simulink model "realimentacao_estados"  (R2022b)
settings: Solver=VariableStepAuto  StartTime=0.0  StopTime=30  RelTol=1e-3
values from neighbouring files (symbols this model uses):
  Cd = ss_d.C    [espacoDiscreto.m]
  Dd = ss_d.D    [espacoDiscreto.m]
  disturbio = 0.24    [espacoDiscreto.m]
  F = ss_d.A    [espacoDiscreto.m]
  H = ss_d.B    [espacoDiscreto.m]
  K_ganhos = place(F,H,[0.8625,0.8325])    [espacoDiscreto.m]
  R = 1.18    [espacoDiscreto.m]
  T0 = 0.203    [espacoDiscreto.m]
settings Model: Creator=coveiro  LastModifiedBy=gusta

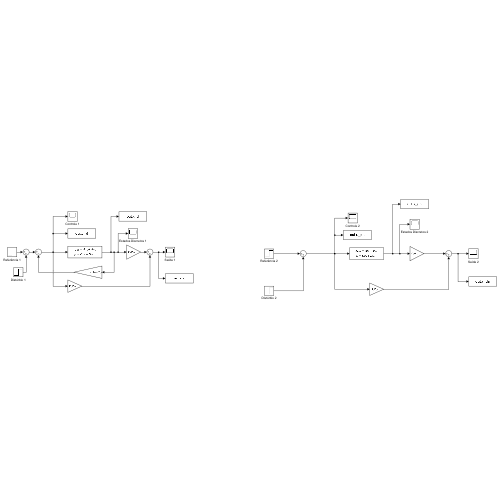
[thumbnail: Simulink's stored preview of the top-level diagram]
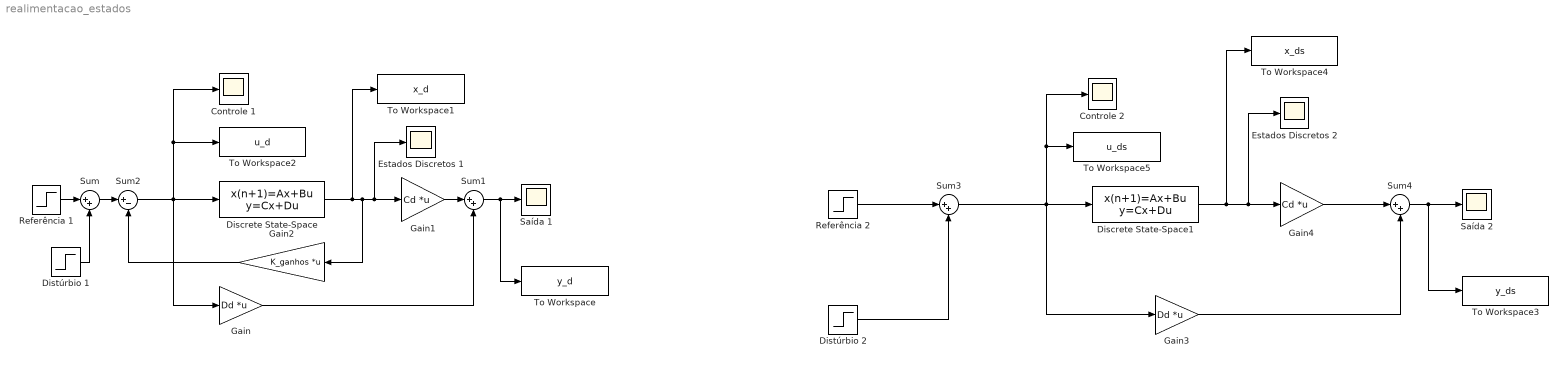
== system realimentacao_estados ==
  Controle 1 : Scope
  Controle 2 : Scope
  Discrete State-Space : DiscreteStateSpace  A=F  B=H  C=[1 0; 0 1]  D=[0;0]  SampleTime=T0
  Discrete State-Space1 : DiscreteStateSpace  A=F  B=H  C=[1 0; 0 1]  D=[0;0]  SampleTime=T0
  Distúrbio 1 : Step  Time=15  After=disturbio  SampleTime=0
  Distúrbio 2 : Step  Time=15  After=disturbio  SampleTime=0
  Estados Discretos 1 : Scope
  Estados Discretos 2 : Scope
  Gain : Gain  Gain=Dd  Multiplication=Matrix(K*u)
  Gain1 : Gain  Gain=Cd  Multiplication=Matrix(K*u)
  Gain2 : Gain  Gain=K_ganhos  Multiplication=Matrix(K*u)
  Gain3 : Gain  Gain=Dd  Multiplication=Matrix(K*u)
  Gain4 : Gain  Gain=Cd  Multiplication=Matrix(K*u)
  Referência 1 : Step  Time=0  After=R  SampleTime=0
  Referência 2 : Step  Time=0  After=R  SampleTime=0
  Saída 1 : Scope
  Saída 2 : Scope
  Sum{,1,3..4} (4 alike) : Sum  Inputs=|++
  Sum2 : Sum  Inputs=|+-
  To Workspace : ToWorkspace  VariableName=y_d  SaveFormat=Timeseries  SampleTime=-1
  To Workspace1 : ToWorkspace  VariableName=x_d  SaveFormat=Timeseries  SampleTime=-1
  To Workspace2 : ToWorkspace  VariableName=u_d  SaveFormat=Timeseries  SampleTime=-1
  To Workspace3 : ToWorkspace  VariableName=y_ds  SaveFormat=Timeseries  SampleTime=-1
  To Workspace4 : ToWorkspace  VariableName=x_ds  SaveFormat=Timeseries  SampleTime=-1
  To Workspace5 : ToWorkspace  VariableName=u_ds  SaveFormat=Timeseries  SampleTime=-1
  wires:
  Discrete State-Space/1 -> To Workspace1/1, Gain2/1, Estados Discretos 1/1, Gain1/1
  Gain/1 -> Sum1/2
  Gain1/1 -> Sum1/1
  Sum1/1 -> To Workspace/1, Saída 1/1
  Sum/1 -> Sum2/1
  Sum2/1 -> Controle 1/1, To Workspace2/1, Gain/1, Discrete State-Space/1
  Referência 1/1 -> Sum/1
  Distúrbio 1/1 -> Sum/2
  Gain2/1 -> Sum2/2
  Sum4/1 -> To Workspace3/1, Saída 2/1
  Referência 2/1 -> Sum3/1
  Sum3/1 -> Controle 2/1, To Workspace5/1, Gain3/1, Discrete State-Space1/1
  Distúrbio 2/1 -> Sum3/2
  Discrete State-Space1/1 -> To Workspace4/1, Estados Discretos 2/1, Gain4/1
  Gain3/1 -> Sum4/2
  Gain4/1 -> Sum4/1
